simulink model "Non_Linear_model"  (R2025b)
settings: Solver=VariableStepAuto  StartTime=0.0  StopTime=20  RelTol=1e-3
InitFcn:
  | load('drone_model_parameters.mat');
values from neighbouring files (symbols this model uses):
  g = 9.81    [drone_model_parameters.m]    (also in drone_model_parameters.mat)
  J11 = 5.8286e-5    (= 5.8286e-05)    [drone_model_parameters.m]    (also in drone_model_parameters.mat)
  J22 = 7.1691e-5    (= 7.1691e-05)    [drone_model_parameters.m]    (also in drone_model_parameters.mat)
  J33 = 3.0e-5    (= 3e-05)    [drone_model_parameters.m]    (also in drone_model_parameters.mat)
  K_T = 4.72e-08    [drone_model_parameters.m]    (also in drone_model_parameters.mat)
  K_tau = 1.1393e-10    [drone_model_parameters.m]    (also in drone_model_parameters.mat)
  K_u = 13840.4    [drone_model_parameters.m]    (also in drone_model_parameters.mat)
  L = 0.0624    [drone_model_parameters.m]    (also in drone_model_parameters.mat)
  m = 0.063    [drone_model_parameters.m]    (also in drone_model_parameters.mat)
  u_imax = 500    [drone_model_parameters.m]    (also in drone_model_parameters.mat)
libraries: matrix_library x1
settings Model: Creator=Lenovo  LastModifiedBy=pepev

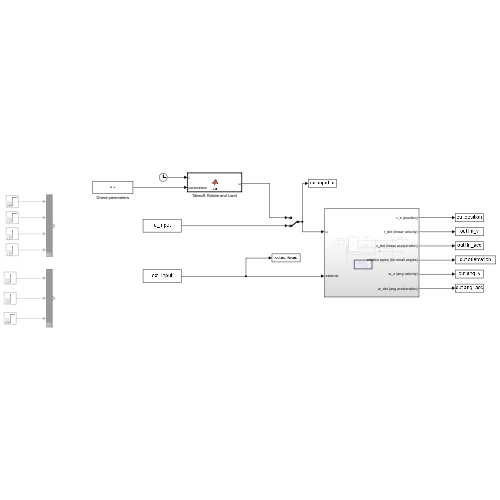
[thumbnail: Simulink's stored preview of the top-level diagram]
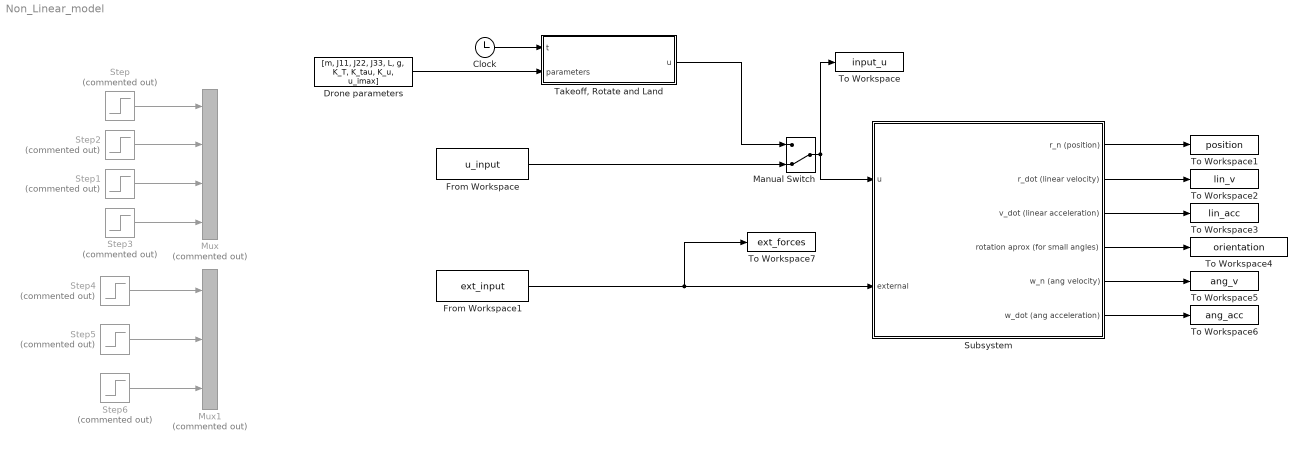
== system Non_Linear_model ==
  Clock : Clock
  Drone parameters : Constant  Value=[m, J11, J22, J33, L, g, K_T, K_tau, K_u, u_imax]
  From Workspace : FromWorkspace  VariableName=u_input  SampleTime=0.01
  From Workspace1 : FromWorkspace  VariableName=ext_input  SampleTime=0.01
  Manual Switch : ManualSwitch  CurrentSetting=0
  Mux : Mux  Commented=on
  Mux1 : Mux  Commented=on  Inputs=3
  Step{,1..6} (7 alike) : Step  Commented=on  SampleTime=0
  Subsystem : Subsystem
  "Takeoff, Rotate and Land" : MATLAB Function  TreatAsAtomicUnit=on
  To Workspace : ToWorkspace  VariableName=input_u  SaveFormat=Timeseries  SampleTime=-1
  To Workspace1 : ToWorkspace  VariableName=position  SaveFormat=Timeseries  SampleTime=-1
  To Workspace2 : ToWorkspace  VariableName=lin_v  SaveFormat=Timeseries  SampleTime=-1
  To Workspace3 : ToWorkspace  VariableName=lin_acc  SaveFormat=Timeseries  SampleTime=-1
  To Workspace4 : ToWorkspace  VariableName=orientation  SaveFormat=Timeseries  SampleTime=-1
  To Workspace5 : ToWorkspace  VariableName=ang_v  SaveFormat=Timeseries  SampleTime=-1
  To Workspace6 : ToWorkspace  VariableName=ang_acc  SaveFormat=Timeseries  SampleTime=-1
  To Workspace7 : ToWorkspace  VariableName=ext_forces  SaveFormat=Timeseries  SampleTime=-1
  wires:
  Subsystem/1(r_n (position)) -> To Workspace1/1
  Step2/1 -> Mux/2
  From Workspace1/1 -> To Workspace7/1, Subsystem/2(external)
  Step1/1 -> Mux/3
  Step3/1 -> Mux/4
  Step4/1 -> Mux1/1
  Step6/1 -> Mux1/3
  Subsystem/2(r_dot (linear velocity)) -> To Workspace2/1
  Subsystem/3(v_dot (linear acceleration)) -> To Workspace3/1
  Subsystem/4(rotation aprox (for small angles)) -> To Workspace4/1
  Subsystem/5(w_n (ang velocity)) -> To Workspace5/1
  Subsystem/6(w_dot (ang acceleration)) -> To Workspace6/1
  "Takeoff, Rotate and Land"/1(u) -> Manual Switch/1
  Manual Switch/1 -> To Workspace/1, Subsystem/1(u)
  Drone parameters/1 -> "Takeoff, Rotate and Land"/2(parameters)
  Clock/1 -> "Takeoff, Rotate and Land"/1(t)
  Step/1 -> Mux/1
  Step5/1 -> Mux1/2
  From Workspace/1 -> Manual Switch/2

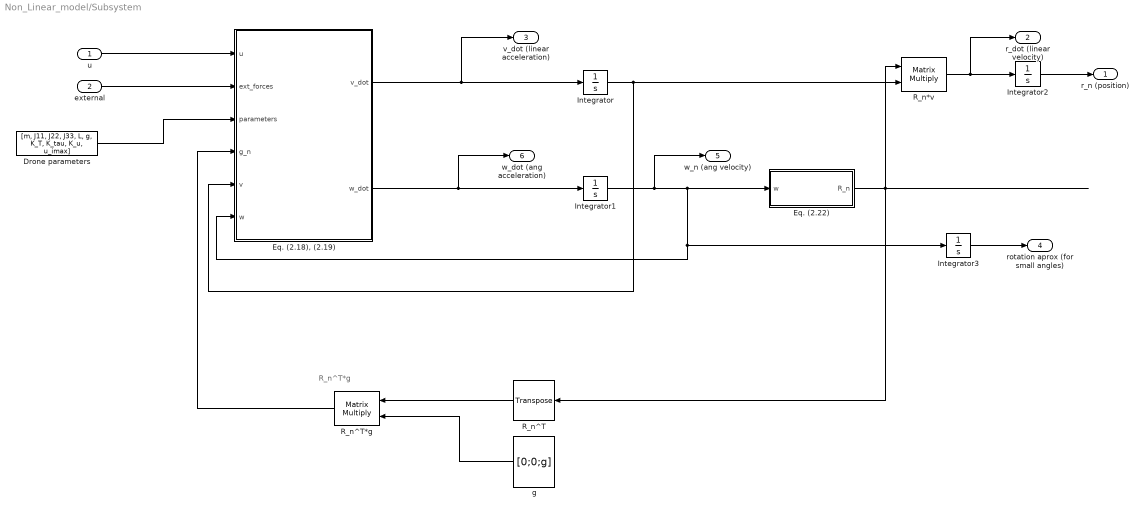
== system Non_Linear_model/Subsystem ==
  note: R_n^T*g
  u : Inport
  external : Inport  Port=2
  Drone parameters : Constant  Value=[m, J11, J22, J33, L, g, K_T, K_tau, K_u, u_imax]
  "Eq. (2.18), (2.19) " : MATLAB Function  TreatAsAtomicUnit=on
  Eq. (2.22) : Subsystem
  Integrator{,1..3} (4 alike) : Integrator
  R_n*v : Product  Multiplication=Matrix(*)
  R_n^T : matrix_library/Transpose
  R_n^T*g : Product  Multiplication=Matrix(*)
  g : Constant  Value=[0;0;g]  VectorParams1D=off
  r_n (position) : Outport
  r_dot (linear velocity) : Outport  Port=2
  v_dot (linear acceleration) : Outport  Port=3
  rotation aprox (for small angles) : Outport  Port=4
  w_n (ang velocity) : Outport  Port=5
  w_dot (ang acceleration) : Outport  Port=6
  wires:
  u/1 -> "Eq. (2.18), (2.19) "/1(u)
  external/1 -> "Eq. (2.18), (2.19) "/2(ext_forces)
  Drone parameters/1 -> "Eq. (2.18), (2.19) "/3(parameters)
  Eq. (2.22)/1(R_n) -> R_n*v/1, R_n^T/1
  R_n*v/1 -> r_dot (linear velocity)/1, Integrator2/1
  Integrator2/1 -> r_n (position)/1
  "Eq. (2.18), (2.19) "/1(v_dot) -> v_dot (linear acceleration)/1, Integrator/1
  "Eq. (2.18), (2.19) "/2(w_dot) -> w_dot (ang acceleration)/1, Integrator1/1
  Integrator/1 -> "Eq. (2.18), (2.19) "/5(v), R_n*v/2
  Integrator1/1 -> w_n (ang velocity)/1, Eq. (2.22)/1(w), "Eq. (2.18), (2.19) "/6(w), Integrator3/1
  Integrator3/1 -> rotation aprox (for small angles)/1
  R_n^T/1 -> R_n^T*g/1
  g/1 -> R_n^T*g/2
  R_n^T*g/1 -> "Eq. (2.18), (2.19) "/4(g_n)

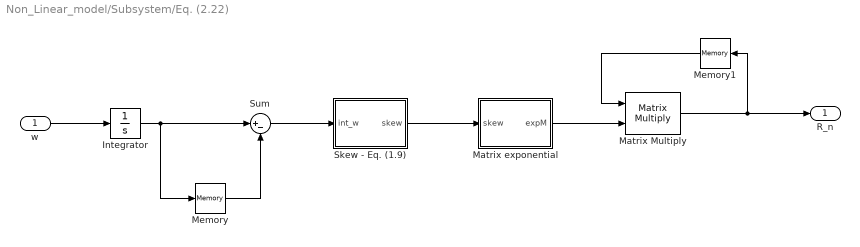
== system Non_Linear_model/Subsystem/Eq. (2.22) ==
  w : Inport
  Integrator : Integrator  InitialCondition=[0;0;0]
  Matrix Multiply : Product  Multiplication=Matrix(*)
  Matrix exponential : MATLAB Function  TreatAsAtomicUnit=on
  Memory : Memory  InitialCondition=[0 0 0]
  Memory1 : Memory  InitialCondition=eye(3)
  Skew - Eq. (1.9) : MATLAB Function  TreatAsAtomicUnit=on
  Sum : Sum  Inputs=|+-
  R_n : Outport
  wires:
  w/1 -> Integrator/1
  Integrator/1 -> Memory/1, Sum/1
  Memory/1 -> Sum/2
  Sum/1 -> Skew - Eq. (1.9)/1(int_w)
  Skew - Eq. (1.9)/1(skew) -> Matrix exponential/1(skew)
  Matrix exponential/1(expM) -> Matrix Multiply/2
  Matrix Multiply/1 -> Memory1/1, R_n/1
  Memory1/1 -> Matrix Multiply/1

== matlab function Non_Linear_model/Subsystem/Eq. (2.22)/Skew - Eq. (1.9) ==
  data: int_w input; skew output
function skew = fcn(int_w)

skew = [0 -int_w(3) int_w(2); int_w(3) 0 -int_w(1); -int_w(2) int_w(1) 0];

end

== matlab function Non_Linear_model/Subsystem/Eq. (2.18), (2.19)  ==
  data: u input; ext_forces input; parameters input; g_n input; v input size=3; w input size=3; v_dot output size=3; w_dot output size=3
function [v_dot, w_dot] = fcn(u, ext_forces, parameters, g_n, v, w)
% Implements Equations 2.18 and 2.19 from the quadcopter dynamics notes
%
% Inputs:
%   u           - control inputs [F3; M1; M2; M3]
%   ext_forces  - external force perturbations [F1ext; F2ext; F3ext] in body frame
%   parameters  - drone parameters [m; J11; J22; J33]
%   g_n         - gravity vector projected in body frame [g1; g2; g3]
%   v           - linear velocity in body frame [v1; v2; v3]
%   w           - angular velocity in body frame [w1; w2; w3]
%
% Outputs:
%   v_dot       - linear acceleration in body frame [v1_dot; v2_dot; v3_dot]
%   w_dot       - angular acceleration in body frame [w1_dot; w2_dot; w3_dot]

% ── Unpack control inputs ─────────────────────────────────────────────────
F3 = u(1);
M1 = u(2);
M2 = u(3);
M3 = u(4);

% ── Unpack external forces ────────────────────────────────────────────────
F1_ext = ext_forces(1);
F2_ext = ext_forces(2);
F3_ext = ext_forces(3);

% ── Unpack parameters ─────────────────────────────────────────────────────
m   = parameters(1);
J11 = parameters(2);
J22 = parameters(3);
J33 = parameters(4);

% ── Linear acceleration - Eq. 2.18 ───────────────────────────────────────
% v_dot = Coriolis + thrust/ext forces + gravity projection
v_dot_1 = (v(2)*w(3) - v(3)*w(2)) + (F1_ext/m) + g_n(1);
v_dot_2 = (v(3)*w(1) - v(1)*w(3)) + (F2_ext/m) + g_n(2);
v_dot_3 = (v(1)*w(2) - v(2)*w(1)) + (F3/m) + (F3_ext/m) + g_n(3);

% ── Angular acceleration - Eq. 2.19 ──────────────────────────────────────
% w_dot = gyroscopic terms + applied moments
w_dot_1 = ((J22-J33)/J11) * w(2)*w(3) + M1/J11;
w_dot_2 = ((J33-J11)/J22) * w(1)*w(3) + M2/J22;
w_dot_3 = ((J11-J22)/J33) * w(1)*w(2) + M3/J33;

% ── Pack outputs ──────────────────────────────────────────────────────────
v_dot = [v_dot_1; v_dot_2; v_dot_3];
w_dot = [w_dot_1; w_dot_2; w_dot_3];

== matlab function Non_Linear_model/Subsystem/Eq. (2.22)/Matrix exponential ==
  data: skew input; expM output
function expM = fcn(skew)

expM = expm(skew);

== matlab function Non_Linear_model/Takeoff, Rotate and Land ==
  data: t input; u output; parameters input
function u = fcn(t, parameters)
% Computes the generalized forces [F3; M1; M2; M3] for the
% Takeoff, Rotate and Land maneuver - Eq. 2.28

% ── Unpack parameters ─────────────────────────────────────────────────────
m   = parameters(1);
% J11 = parameters(2);  % not needed here (M1=0)
% J22 = parameters(3);  % not needed here (M2=0)
J33 = parameters(4);
% L   = parameters(5);  % not needed here
g   = parameters(6);

% ── Maneuver time intervals and acceleration magnitudes ───────────────────
t_to   = 5;       % Takeoff duration [s]
t_rot  = 10;      % Rotation duration [s]
t_land = 5;       % Landing duration [s]

alfa_to   = -0.016;  % Takeoff acceleration magnitude [m/s^2]
alfa_rot  = pi/25;   % Rotation acceleration magnitude [rad/s^2]
alfa_land =  0.016;  % Landing acceleration magnitude [m/s^2]

% ── Piecewise constant acceleration profile - Eq. 2.23 ───────────────────
    function q_ddot = acceleration(alfa, tf, t)
        if t >= 0 && t < tf/2
            q_ddot = alfa;
        elseif t >= tf/2 && t <= tf
            q_ddot = -alfa;
        else
            q_ddot = 0;
        end
    end

% ── Generalized forces - Eq. 2.28 ────────────────────────────────────────
F3 = m*acceleration(alfa_to, t_to, t) + ...
     m*acceleration(alfa_land, t_land, t-t_to-t_rot) - m*g;
M1 = 0;
M2 = 0;
M3 = J33 * acceleration(alfa_rot, t_rot, t-t_to);

u = [F3; M1; M2; M3];
end
